simulink model "mainSimulink_localPi"  (R2021a)
settings: Solver=VariableStepAuto  StartTime=0.0  StopTime=20  FixedStep=samplingTime  RelTol=1e-3
model workspace (MATLAB code in the model file):
  | %% Simulink settings
  | controllerFile = 'directFFcontroller';
  | set_param('mainSimulink_localPi/Subsystem Reference', 'ReferencedSubsystem', controllerFile);
  | %% Display settings
  | scopeTimeSpan = 30;
  | 
  | %% Robot settings (must match Python)
  | sensorFreq = 125;
  | actuatorFreq = 250;
  | TCPport = 12345;
  | dataSize = 1;
  | sensorSamplingTime = 1/sensorFreq;
  | actuatorTime = 1/actuatorFreq;
undefined symbols (not defined in the file): f
libraries: instrumentlib x2
settings Model: Creator=chukh  LastModifiedBy=brandon

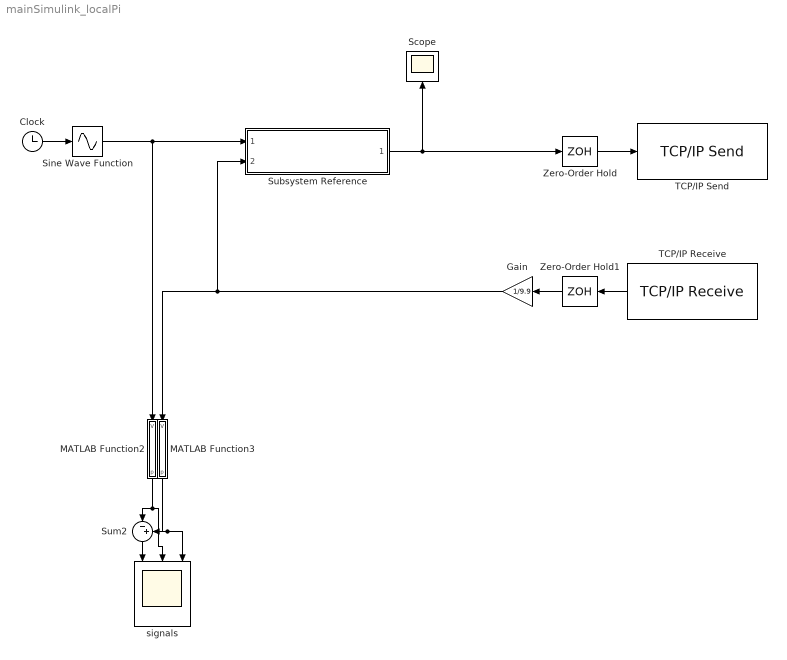
== system mainSimulink_localPi ==
  Clock : Clock
  Gain : Gain  Gain=1/9.9
  MATLAB Function2 : MATLAB Function  TreatAsAtomicUnit=on
  MATLAB Function3 : MATLAB Function  TreatAsAtomicUnit=on
  Scope : Scope
  Sine Wave Function : Sin  TimeSource=Use external signal  Amplitude=.2  Bias=0.6  Frequency=2  SampleTime=0
  Subsystem Reference : Subsystem  ReferencedSubsystem=directFFcontroller
  Sum2 : Sum  Inputs=|-+
  TCP/IP Receive : instrumentlib/TCP//IP Receive  Host=server.softrobot  Port=TCPport  DataSize=dataSize  EnableBlockingMode=on  Timeout=0.5  SampleTime=sensorSamplingTime  DataType=double  ByteOrder=LittleEndian  ASCIIFormatting=%f,  Terminator=LF
  TCP/IP Send : instrumentlib/TCP//IP Send  Host=server.softrobot  Port=TCPport  EnableBlockingMode=on  Timeout=0.5  ByteOrder=LittleEndian  TransferDelay=on
  Zero-Order Hold : ZeroOrderHold  SampleTime=actuatorTime
  Zero-Order Hold1 : ZeroOrderHold  SampleTime=actuatorTime
  signals : Scope  NumInputPorts=3
  wires:
  Subsystem Reference/1 -> Zero-Order Hold/1, Scope/1
  TCP/IP Receive/1 -> Zero-Order Hold1/1
  Zero-Order Hold/1 -> TCP/IP Send/1
  Zero-Order Hold1/1 -> Gain/1
  MATLAB Function2/1(p) -> Sum2/1, signals/2
  Gain/1 -> MATLAB Function3/1(V), Subsystem Reference/2
  MATLAB Function3/1(p) -> Sum2/2, signals/3
  Sine Wave Function/1 -> Subsystem Reference/1, MATLAB Function2/1(V)
  Sum2/1 -> signals/1
  Clock/1 -> Sine Wave Function/1

== matlab function mainSimulink_localPi/MATLAB Function3 ==
  data: V input; p output
function p = V2kPa(V)
p = (V-0.5)*200;

== matlab function mainSimulink_localPi/MATLAB Function2 ==
  data: V input; p output
function p = V2kPa(V)
p = (V-0.5)*200;
